simulink model "test_Mixer_Pt1"  (R2018b)
settings: Solver=ode45  StartTime=0.0  StopTime=6000  FixedStep=5
undefined symbols (not defined in the file): path_carnot
libraries: carnot x9, simulink x4, simulink_extras x1
Description:
  | % This file is part of the CARNOT Blockset.
  | %
  | % Copyright (c) 1998-2015, Solar-Institute Juelich of the FH Aachen.
  | % Additional Copyright for this file see list auf authors.
  | % All rights reserved.
  | %
  | % Redistribution and use in source and binary forms, with or without
  | % modification, are permitted provided that the following conditions are
  | % met:
  | %
  | % 1. Redistributions of source code must retain the above copyright notice,
  | %    this list of conditions and the following disclaimer.
  | %
  | % 2. Redistributions in binary form must reproduce the above copyright
  | %    notice, this list of conditions and the following disclaimer in the
  | %    documentation and/or other materials provided with the distribution.
  | %
  | % 3. Neither the name of the copyright holder nor the names of its
  | %    contributors may be used to endorse or promote products derived from
  | %    this software without specific prior written permission.
  | %
  | % THIS SOFTWARE IS PROVIDED BY THE COPYRIGHT HOLDERS AND CONTRIBUTORS "AS IS"
  | % AND ANY EXPRESS OR IMPLIED WARRANTIES, INCLUDING, BUT NOT LIMITED TO, THE
  | % IMPLIED WARRANTIES OF MERCHANTABILITY AND FITNESS FOR A PARTICULAR PURPOSE
  | % ARE DISCLAIMED. IN NO EVENT SHALL THE COPYRIGHT HOLDER OR CONTRIBUTORS BE
  | % LIABLE FOR ANY DIRECT, INDIRECT, INCIDENTAL, SPECIAL, EXEMPLARY, OR
  | % CONSEQUENTIAL DAMAGES (INCLUDING, BUT NOT LIMITED TO, PROCUREMENT OF
  | % SUBSTITUTE GOODS OR SERVICES; LOSS OF USE, DATA, OR PROFITS; OR BUSINESS
  | % INTERRUPTION) HOWEVER CAUSED AND ON ANY THEORY OF LIABILITY, WHETHER IN
  | % CONTRACT, STRICT LIABILITY, OR TORT (INCLUDING NEGLIGENCE OR OTHERWISE)
  | % ARISING IN ANY WAY OUT OF THE USE OF THIS SOFTWARE, EVEN IF ADVISED OF
  | % THE POSSIBILITY OF SUCH DAMAGE.
settings Model: ExtModeTrigMode=oneshot  ExtModeArmWhenConnect=off  Creator=FarG  LastModifiedBy=drhf
settings Model: ModifiedHistory=|
  | Created by Gaelle Faure
  | Revised by Bernd Hafner
settings SolverCC: MaxOrder=3  ZeroCrossControl=DisableAll
settings DataIOCC: SaveFormat=Array  SaveOutput=off  SaveTime=off  ReturnWorkspaceOutputs=on
settings OptimizationCC: DefaultParameterBehavior=Inlined  ExpressionDepthLimit=2147483647  InitFltsAndDblsToZero=on  LifeSpan=inf
settings DebuggingCC: ReadBeforeWriteMsg=DisableAll  WriteAfterWriteMsg=DisableAll  WriteAfterReadMsg=DisableAll  SaveWithParameterizedLinksMsg=none  UnderspecifiedInitializationDetection=Classic  MergeDetectMultiDrivingBlocksExec=none  MultiTaskDSMMsg=none  MultiTaskCondExecSysMsg=none  StateNameClashWarn=warning  SFUnexpectedBacktrackingDiag=warning  SFNoUnconditionalDefaultTransitionDiag=warning  SFExecutionAtInitializationDiag=none
settings HardwareCC: ProdBitPerPointer=32  ProdBitPerSizeT=32  ProdBitPerPtrDiffT=32  ProdLargestAtomicFloat=None  ProdIntDivRoundTo=Undefined  ProdEndianess=Unspecified  ProdWordSize=32  ProdHWDeviceType=32-bit Generic  TargetUnknown=on
settings ModelReferenceCC: UpdateModelReferenceTargets=IfOutOfDate  PropagateSignalLabelsOutOfModel=off
settings SFSimCC: SFSimEcho=off  SimUseLocalCustomCode=off
settings RTWCC: RTWUseLocalCustomCode=off
settings CodeAppCC: StateflowObjectComments=on
settings GRTTargetCC: TargetFcnLib=ansi_tfl_tmw.mat  TargetLangStandard=C89/C90 (ANSI)  ModelReferenceCompliant=off  ParMdlRefBuildCompliant=off  CompOptLevelCompliant=off  GeneratePreprocessorConditionals=Disable all  CombineOutputUpdateFcns=off  MatFileLogging=off  GRTInterface=on
settings ConfigComp: CovMetricSettings=dw  CovHtmlReporting=on  CovSaveCumulativeToWorkspaceVar=on  CovSaveSingleToWorkspaceVar=on  CovExternalEMLEnable=off

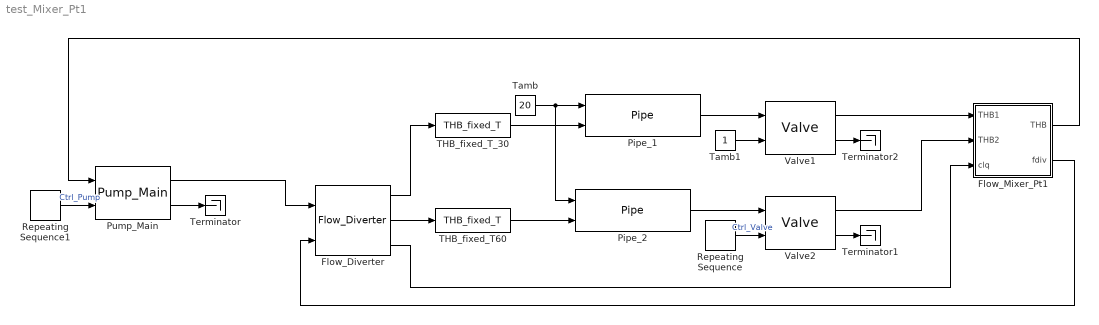
== system test_Mixer_Pt1 ==
  Flow_Diverter : carnot/Hydraulics/Flow_Diverter
  Flow_Mixer_Pt1 : Subsystem  mask(flow mixer){t_fdiv=10}
      mask prompts: t_fdiv "Time constant of the mixer in s"
      mask help: Mixes two massflows. The new temperature is calculated by an energy balance. The output f_div may be fed back to the corresponding flow diverter upwards in flowdirection.
      mask Help: web(fullfile(path_carnot('help'),'Flow_Mixer.html'),'-helpbrowser')
      mask TypeOptions t_fdiv: PT1_for_fdiv/t_fdiv
      mask Display: plot(-25,-5,95,65,[20 45 20 20],[20 30 40 20],[45 70 70 45],[30 20 40 30],[45 35 55 45],[30 10 10 30])
  Pipe_1 : carnot/Hydraulics/Pipe  dia=0.02  len=10  hgt=5  uloss=100/20/10  cond=0  cwall=1000  t0=20  lin=100/0.2  qua=100/0.2^2  nodes=10
  Pipe_2 : carnot/Hydraulics/Pipe  dia=0.02  len=10  hgt=5  uloss=100/20/10  cond=0  cwall=1000  t0=20  lin=100/0.2  qua=100/0.2^2  nodes=10
  Pump_Main : carnot/Hydraulics/Pump_Main  Tini=20  p0=3e5  IDpreset=pressure drop  fluid=Water  mix=0  mix2=0  mix3=0  t1=5  PathName=fullfile(path_carnot('libsl'), 'Hydraulics', 'Pump_Main', 'parameter_set')  FileName='Pump6m.mat'  userPath=off  userParam=off  a0=60000  a1=-43200  a2=0  dia=0.025  UA=1  mcp=4182  e0=50  e1=28.8  e2=-10.368
  Repeating Sequence : simulink/Sources/Repeating Sequence  rep_seq_t=[0 100 180 200]  rep_seq_y=[1 1 0 0]
  Repeating Sequence1 : simulink/Sources/Repeating Sequence  rep_seq_t=[ 0 300 300+eps(300) 400 400+eps(400) 600]  rep_seq_y=[ 1 1 0+0*eps(300) 0 1+0*eps(400) 1]
  THB_fixed_T60 : carnot/Source/Simple/THB_fixed_T  t=60
  THB_fixed_T_30 : carnot/Source/Simple/THB_fixed_T  t=30
  Tamb : Constant  Value=20
  Tamb1 : Constant
  Terminator : Terminator
  Terminator1 : Terminator
  Terminator2 : Terminator
  Valve1 : carnot/Hydraulics/Valve  vtyp=linear  psi_0=0.04  kvs=0.2*3600/1000  dt_V=30
  Valve2 : carnot/Hydraulics/Valve  vtyp=linear  psi_0=0.04  kvs=0.2*3600/1000  dt_V=30
  wires:
  Flow_Diverter/1 -> THB_fixed_T_30/1
  Tamb/1 -> Pipe_1/1, Pipe_2/1
  Flow_Diverter/2 -> THB_fixed_T60/1
  Pipe_2/1 -> Valve2/1
  Repeating Sequence/1 -> Valve2/2  "Ctrl_Valve"
  Valve2/1 -> Flow_Mixer_Pt1/2(THB2)
  Repeating Sequence1/1 -> Pump_Main/2  "Ctrl_Pump"
  Pump_Main/2 -> Terminator/1
  Pump_Main/1 -> Flow_Diverter/1
  Flow_Mixer_Pt1/1(THB) -> Pump_Main/1
  Valve1/1 -> Flow_Mixer_Pt1/1(THB1)
  Flow_Diverter/3 -> Flow_Mixer_Pt1/3(clq)
  Flow_Mixer_Pt1/2(fdiv) -> Flow_Diverter/2
  THB_fixed_T_30/1 -> Pipe_1/2
  THB_fixed_T60/1 -> Pipe_2/2
  Valve2/2 -> Terminator1/1
  Pipe_1/1 -> Valve1/1
  Tamb1/1 -> Valve1/2
  Valve1/2 -> Terminator2/1

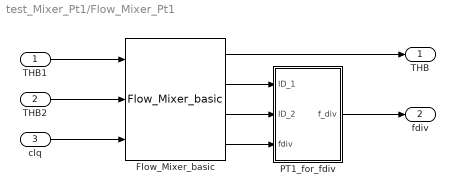
== system test_Mixer_Pt1/Flow_Mixer_Pt1 ==
  THB1 : Inport
  THB2 : Inport  Port=2
  clq : Inport  Port=3
  Flow_Mixer_basic : carnot/Basic/Hydraulics/Flow_Mixer_basic
  PT1_for_fdiv : Subsystem  mask{t_fdiv=t_fdiv}
      mask prompts: t_fdiv "Time constant for fdiv in s"
  THB : Outport
  fdiv : Outport  Port=2
  wires:
  clq/1 -> Flow_Mixer_basic/3
  PT1_for_fdiv/1(f_div) -> fdiv/1
  THB1/1 -> Flow_Mixer_basic/1
  THB2/1 -> Flow_Mixer_basic/2
  Flow_Mixer_basic/1 -> THB/1
  Flow_Mixer_basic/2 -> PT1_for_fdiv/1(ID_1)
  Flow_Mixer_basic/3 -> PT1_for_fdiv/2(ID_2)
  Flow_Mixer_basic/4 -> PT1_for_fdiv/3(fdiv)

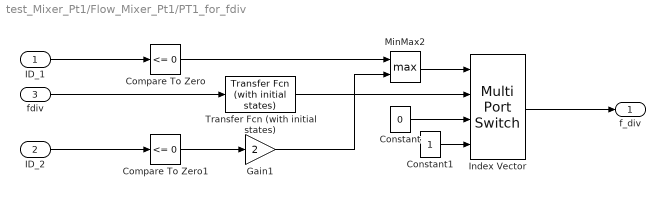
== system test_Mixer_Pt1/Flow_Mixer_Pt1/PT1_for_fdiv ==
  ID_1 : Inport
  ID_2 : Inport  Port=2
  fdiv : Inport  Port=3
  Compare To Zero : simulink/Logic and Bit Operations/Compare To Zero  relop=<=  OutDataTypeStr=uint8
  Compare To Zero1 : simulink/Logic and Bit Operations/Compare To Zero  relop=<=  OutDataTypeStr=uint8
  Constant : Constant  Value=0
  Constant1 : Constant
  Gain1 : Gain  Gain=2
  Index Vector : MultiPortSwitch  DataPortOrder=Zero-based contiguous  zeroidx=on
  MinMax2 : MinMax  Function=max  Inputs=2
  Transfer Fcn (with initial states) : simulink_extras/Additional Linear/Transfer Fcn (with initial states)  N=[1]  D="[t_fdiv  1]"  X0=0.5*t_fdiv
  f_div : Outport
  wires:
  fdiv/1 -> Transfer Fcn (with initial states)/1
  Compare To Zero1/1 -> Gain1/1
  Compare To Zero/1 -> MinMax2/1
  MinMax2/1 -> Index Vector/1
  ID_1/1 -> Compare To Zero/1
  ID_2/1 -> Compare To Zero1/1
  Constant/1 -> Index Vector/3
  Transfer Fcn (with initial states)/1 -> Index Vector/2
  Constant1/1 -> Index Vector/4
  Gain1/1 -> MinMax2/2
  Index Vector/1 -> f_div/1
